simulink model "Buck_converter_Lab"  (R2025a)
settings: Solver=ode23tb  StartTime=0.0  StopTime=0.1  RelTol=1e-3
values from neighbouring files (symbols this model uses):
  C = 220e-6    (= 0.00022)    [load_parameters.m]
  d = 0.5    [load_parameters.m]
  f = 5000    [load_parameters.m]
  L = 800e-6    (= 0.0008)    [load_parameters.m]
  R = 7    [load_parameters.m]
  Vin = 14    [load_parameters.m]
libraries: spsParallelRLCBranchLib x6, spsCurrentMeasurementLib x5, spsMeanLib x4, spsDCVoltageSourceLib x2, spsDiodeLib x2, spsGroundLib x2, spsMosfetLib x2, spsVoltageMeasurementLib x2, sps_lib x1
settings Model: Creator=ashka  LastModifiedBy=Mads2
settings SolverCC: AlgebraicLoopSolver=TrustRegion
settings DebuggingCC: UnconnectedInputMsg=warning  UnconnectedOutputMsg=warning  UnconnectedLineMsg=warning
settings ModelReferenceCC: EnableRefExpFcnMdlSchedulingChecks=on
settings RTWCC: GPUComputeCapability=3.5  DLArmComputeVersion=19.05

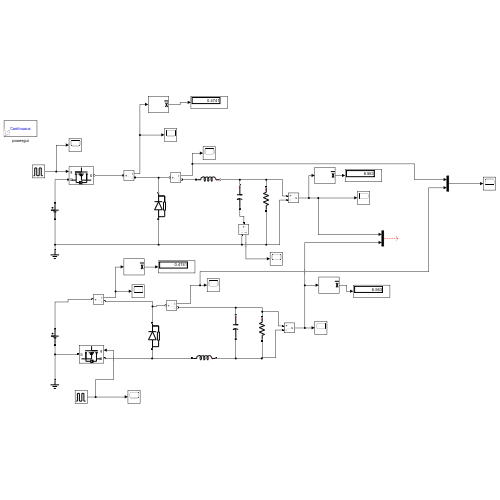
[thumbnail: Simulink's stored preview of the top-level diagram]
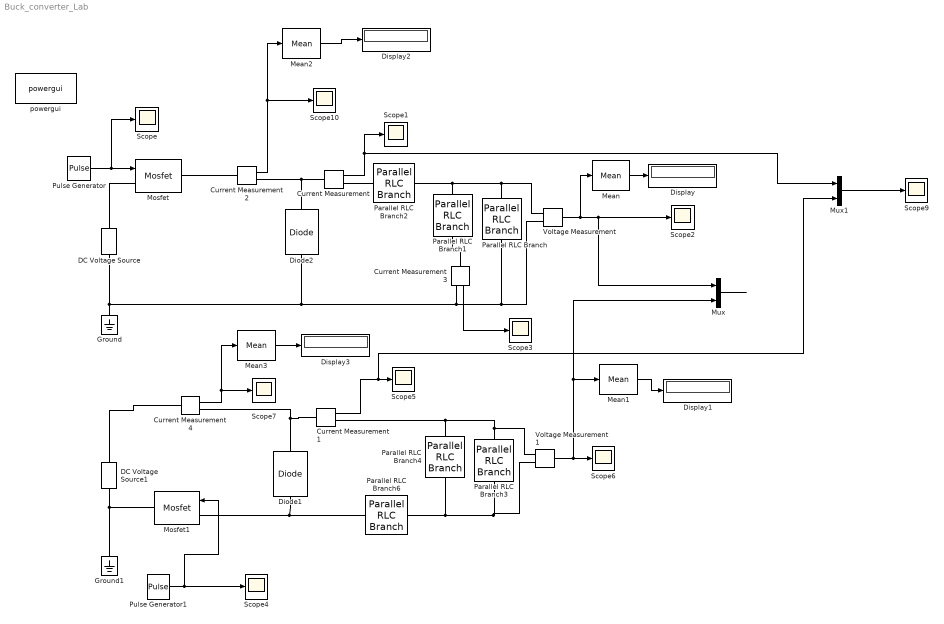
== system Buck_converter_Lab ==
  Current Measurement{,1..4} (5 alike) : spsCurrentMeasurementLib/Current Measurement  PhasorSimulation=off  OutputType=Complex  PSBequivalent=0
  DC Voltage Source : spsDCVoltageSourceLib/DC Voltage Source  Amplitude=Vin  Measurements=None
  DC Voltage Source1 : spsDCVoltageSourceLib/DC Voltage Source  Amplitude=Vin  Measurements=None
  Diode1 : spsDiodeLib/Diode  Ron=0.001  Lon=0  Vf=0.8  IC=0  UseSnubber=0  Rs=500  Cs=250e-9  Measurements=off
  Diode2 : spsDiodeLib/Diode  Ron=0.001  Lon=0  Vf=0.8  IC=0  UseSnubber=0  Rs=500  Cs=250e-9  Measurements=off
  Display{,1..3} (4 alike) : Display
  Ground : spsGroundLib/Ground  LConnTagsString=a
  Ground1 : spsGroundLib/Ground  LConnTagsString=a
  Mean : spsMeanLib/Mean  Freq=f  Vinit=0  Ts=0
  Mean1 : spsMeanLib/Mean  Freq=f  Vinit=7  Ts=0
  Mean2 : spsMeanLib/Mean  Freq=f  Vinit=0  Ts=0
  Mean3 : spsMeanLib/Mean  Freq=f  Vinit=0  Ts=0
  Mosfet : spsMosfetLib/Mosfet  Ron=0.1  Lon=0  Rd=0.01  Vfd=0  IC=0  Rs=1e5  Cs=inf  Measurements=off
  Mosfet1 : spsMosfetLib/Mosfet  Ron=0.1  Lon=0  Rd=0.01  Vfd=0  IC=0  Rs=1e5  Cs=inf  Measurements=off
  Mux : Mux  Inputs=2
  Mux1 : Mux  Inputs=2
  Parallel RLC Branch : spsParallelRLCBranchLib/Parallel RLC Branch  LConnTagsString=a  RConnTagsString=__new0  BranchType=R  Resistance=R  Inductance=10e-3  SetiL0=off  InitialCurrent=0  Capacitance=1e-6  Setx0=off  InitialVoltage=0  Measurements=None
  Parallel RLC Branch1 : spsParallelRLCBranchLib/Parallel RLC Branch  LConnTagsString=a  RConnTagsString=__new0  BranchType=C  Resistance=10  Inductance=1e-3  SetiL0=off  InitialCurrent=0  Capacitance=C  Setx0=off  InitialVoltage=0  Measurements=None
  Parallel RLC Branch2 : spsParallelRLCBranchLib/Parallel RLC Branch  LConnTagsString=a  RConnTagsString=__new0  BranchType=L  Resistance=10  Inductance=L  SetiL0=off  InitialCurrent=0  Capacitance=1e-6  Setx0=off  InitialVoltage=0  Measurements=None
  Parallel RLC Branch3 : spsParallelRLCBranchLib/Parallel RLC Branch  LConnTagsString=a  RConnTagsString=__new0  BranchType=R  Resistance=R  Inductance=10e-3  SetiL0=off  InitialCurrent=0  Capacitance=1e-6  Setx0=off  InitialVoltage=0  Measurements=None
  Parallel RLC Branch4 : spsParallelRLCBranchLib/Parallel RLC Branch  LConnTagsString=a  RConnTagsString=__new0  BranchType=C  Resistance=10  Inductance=1e-3  SetiL0=off  InitialCurrent=0  Capacitance=C  Setx0=off  InitialVoltage=0  Measurements=None
  Parallel RLC Branch6 : spsParallelRLCBranchLib/Parallel RLC Branch  LConnTagsString=a  RConnTagsString=__new0  BranchType=L  Resistance=10  Inductance=L  SetiL0=off  InitialCurrent=0  Capacitance=1e-6  Setx0=off  InitialVoltage=0  Measurements=None
  Pulse Generator : DiscretePulseGenerator  PulseType=Time based  Amplitude=10  Period=1/f  PulseWidth=d*100
  Pulse Generator1 : DiscretePulseGenerator  PulseType=Time based  Amplitude=10  Period=1/f  PulseWidth=d*100
  Scope{,1..7,9..10} (10 alike) : Scope
      Scope settings: ActiveDisplayYMinimum=2.5277426320283136  ActiveDisplayYMaximum=6.378088127936965
      Scope1 settings: ActiveDisplayYMinimum=-0.79234  ActiveDisplayYMaximum=7.05307
      Scope10 settings: ActiveDisplayYMinimum=-11.94461  ActiveDisplayYMaximum=22.21264
      Scope2 settings: ActiveDisplayYMinimum=-1.55491  ActiveDisplayYMaximum=13.99419  DataLoggingVariableName=ScopeData2
      Scope3 settings: ActiveDisplayYMinimum=-11.94448  ActiveDisplayYMaximum=22.21145  DataLoggingVariableName=ScopeData2
      Scope4 settings: ActiveDisplayYMinimum=-0.625  ActiveDisplayYMaximum=5.625
      Scope5 settings: ActiveDisplayYMinimum=1.50189  ActiveDisplayYMaximum=2.02875  DataLoggingVariableName=ScopeData2
      Scope6 settings: ActiveDisplayYMinimum=12.35956  ActiveDisplayYMaximum=12.36388  DataLoggingVariableName=ScopeData3
      Scope7 settings: ActiveDisplayYMinimum=-11.94461  ActiveDisplayYMaximum=22.21264  DataLoggingVariableName=ScopeData3
      Scope9 settings: ActiveDisplayYMinimum=-0.16501  ActiveDisplayYMaximum=1.46395  DataLoggingVariableName=ScopeData6
  Voltage Measurement : spsVoltageMeasurementLib/Voltage Measurement  PhasorSimulation=off  OutputType=Complex  PSBequivalent=0
  Voltage Measurement1 : spsVoltageMeasurementLib/Voltage Measurement  PhasorSimulation=off  OutputType=Complex  PSBequivalent=0
  powergui : sps_lib/powergui  Priority=1  SimulationMode=Continuous  SampleTime=50e-6  frequency=60  Iterations=50  frequencyindice=0  Pbase=100e6  ErrMax=1e-4  UnitsV=kV  UnitsW=MW  buscounter=0  FunctionMessages=off  echomessages=off  EnableUseOfTLC=off  CurrentSourceSwitches=off  DisableSnubberDevices=off  DisableRonSwitches=off  DisableVfSwitches=off  DisplayEquations=off  AutomaticDiscreteSolvers=off  SolverType=Tustin/Backward Euler (TBE)  Interpol=off  ExternalGateDelay=off  methode=off  Ts=100  x0status=blocks  SPID=on  SwTol=0  HookPort=off  NonlinearTolerance=1e-4  nMaxIteration=100  ContinueOnMaxIteration=off  RestoreLinks=warning  ResistiveCurrentMeasurement=off  Frange=[0:2:500]  Ylog=off  Xlog=on  ShowGrid=off  save=off  variable=ZData  structure=0  ZoomFFT=off  StartTime=0.0  cycles=1  DisplayStyle=1  fundamental=60  FreqAxis=off  MaxFrequency=1000  frequencyindicesteady=1  RmsSteady=1  display=off
  wires:
  Pulse Generator/1 -> Mosfet/1, Scope/1
  Current Measurement/1 -> Scope1/1, Mux1/1
  Mean/1 -> Display/1
  Voltage Measurement/1 -> Mux/1, Scope2/1, Mean/1
  Mean1/1 -> Display1/1
  Current Measurement1/1 -> Mux1/2, Scope5/1
  Pulse Generator1/1 -> Mosfet1/1, Scope4/1
  Voltage Measurement1/1 -> Scope6/1, Mux/2, Mean1/1
  Mux/1 -> ?
  Mux1/1 -> Scope9/1
  Current Measurement2/1 -> Mean2/1, Scope10/1
  Mean2/1 -> Display2/1
  Current Measurement3/1 -> Scope3/1
  Current Measurement4/1 -> Mean3/1, Scope7/1
  Mean3/1 -> Display3/1
  connections:
  Mosfet/LConn1 -- DC Voltage Source/RConn1
  Ground/LConn1 -- DC Voltage Source/LConn1 -- Current Measurement3/RConn1 -- Parallel RLC Branch/RConn1 -- Voltage Measurement/LConn2 -- Diode2/LConn1
  Diode2/RConn1 -- Current Measurement/LConn1 -- Current Measurement2/RConn1
  Parallel RLC Branch2/LConn1 -- Parallel RLC Branch/LConn1 -- Voltage Measurement/LConn1 -- Parallel RLC Branch1/LConn1
  Current Measurement/RConn1 -- Parallel RLC Branch2/RConn1
  Parallel RLC Branch6/RConn1 -- Diode1/LConn1 -- Mosfet1/LConn1
  Diode1/RConn1 -- Current Measurement4/RConn1 -- Current Measurement1/LConn1
  Parallel RLC Branch3/LConn1 -- Voltage Measurement1/LConn1 -- Current Measurement1/RConn1 -- Parallel RLC Branch4/LConn1
  Ground1/LConn1 -- Mosfet1/RConn1 -- DC Voltage Source1/LConn1
  Voltage Measurement1/LConn2 -- Parallel RLC Branch3/RConn1 -- Parallel RLC Branch6/LConn1 -- Parallel RLC Branch4/RConn1
  Mosfet/RConn1 -- Current Measurement2/LConn1
  Parallel RLC Branch1/RConn1 -- Current Measurement3/LConn1
  DC Voltage Source1/RConn1 -- Current Measurement4/LConn1
